simulink model "Demo1_P1C5B"  (R2025b)
settings: Solver=VariableStepAuto  StartTime=0.0  StopTime=3  RelTol=1e-3
settings Model: Creator=abadirwahba  LastModifiedBy=abadirwahba

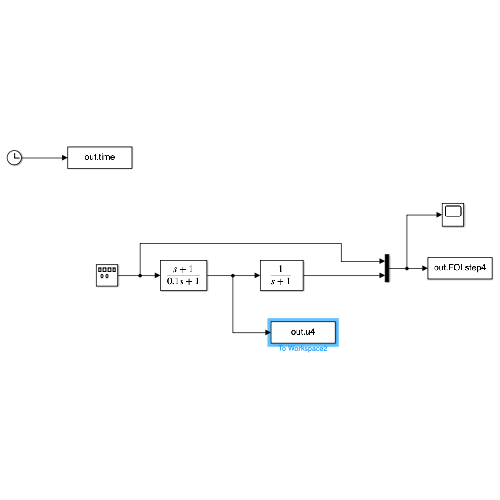
[thumbnail: Simulink's stored preview of the top-level diagram]
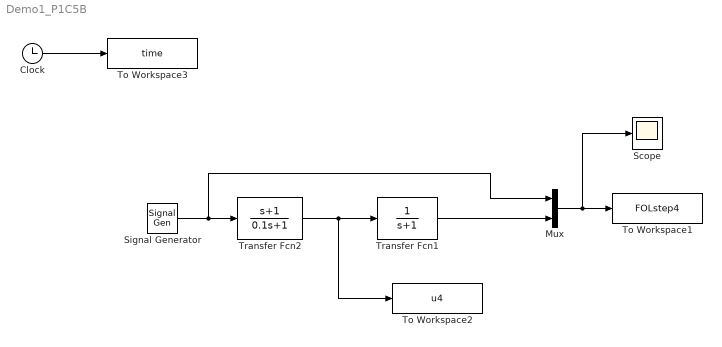
== system Demo1_P1C5B ==
  Clock : Clock
  Mux : Mux  Inputs=2
  Scope : Scope
      settings: ActiveDisplayYMinimum=-1.3475088933434074  ActiveDisplayYMaximum=1.2608343214826008
  Signal Generator : SignalGenerator  WaveForm=square  Frequency=0.5
  To Workspace1 : ToWorkspace  VariableName=FOLstep4  SampleTime=-1
  To Workspace2 : ToWorkspace  VariableName=u4  SampleTime=-1
  To Workspace3 : ToWorkspace  VariableName=time  SampleTime=-1
  Transfer Fcn1 : TransferFcn  Denominator=[1 1]
  Transfer Fcn2 : TransferFcn  Numerator=[1 1]  Denominator=[0.1 1]
  wires:
  Clock/1 -> To Workspace3/1
  Signal Generator/1 -> Transfer Fcn2/1, Mux/1
  Mux/1 -> Scope/1, To Workspace1/1
  Transfer Fcn2/1 -> To Workspace2/1, Transfer Fcn1/1
  Transfer Fcn1/1 -> Mux/2
